simulink model "Katex_FullCar_R2017b_V03"  (R2026a)
settings: Solver=ode1  StopTime=1000  FixedStep=Ts  EnableMultiTasking=on
PostLoadFcn:
  | , if any(exist('dsrtsu_mdlpostloadfcn', 'file') == [2, 3, 6]), try dsrtsu_mdlpostloadfcn('Execute', bdroot); catch fprintf('Error in PostLoadFcn (dsrtsu_mdlpostloadfcn) for model "%s":\n %s\n', bdroot, lasterr); end, end,
  | , if any(exist('dsrtsu_mdlpostloadfcn', 'file') ~= 0), dsrtsu_mdlpostloadfcn('Execute', bdroot); end,
InitFcn:
  | , if any(exist('rtifpga_mdlclblib', 'file') ~= 0), rtifpga_mdlclblib('Init', bdroot); end,
  | 
  | 
  | init
undefined symbols (not defined in the file): locklim_sus, roundN, Ts
libraries: sl_discontinuities x29, simulink_extras x26, simulink x22, mjLib x1
(part 9 of 10)

== system Katex_FullCar_R2017b_V03/DGIST/_Low_Level_Ctrl/Steering_Low_Level_Controller/Torque Mode/Steering Motor Control3/Lag compensator(zeta)/Dot1 ==
  note: Dot
  in : Inport
  Sum1 : Sum  Inputs=+-  InputSameDT=on  SaturateOnIntegerOverflow=on  OutDataTypeStr=Inherit: Same as first input
  Sum2 : Sum  Inputs=+-  InputSameDT=on  SaturateOnIntegerOverflow=on  OutDataTypeStr=Inherit: Same as first input
  d : UnitDelay  SampleTime=Ts
  d1 : UnitDelay  SampleTime=Ts
  gain : Gain  Gain=2/Ts  SaturateOnIntegerOverflow=on  OutDataTypeStr=Inherit: Same as input  ParamDataTypeStr=Inherit: Same as input
  out : Outport  VectorParamsAs1DForOutWhenUnconnected=off
  wires:
  Sum1/1 -> d1/1, out/1
  d1/1 -> Sum1/2
  Sum2/1 -> gain/1
  in/1 -> d/1, Sum2/1
  d/1 -> Sum2/2
  gain/1 -> Sum1/1

== system Katex_FullCar_R2017b_V03/DGIST/_Low_Level_Ctrl/Steering_Low_Level_Controller/Torque Mode/Steering Motor Control3/Lag compensator(zeta)/a//(s+p) ==
  note: y(n) = [(2-p*Ts)*y(n-1)+a*Ts(u(n)+u(n-1))]/(2+p*Ts)
  note: H(s) = a/(s+p)
  note: s = 2/Ts*(z-1)/(z+1)
  In : Inport
  a : Inport  Port=2
  p : Inport  Port=3
  Constant : Constant  Value=2  SampleTime=Ts
  Product1 : Product  Inputs=*/  RndMeth=Zero
  Product11 : Product  RndMeth=Zero
  Product3 : Product  RndMeth=Zero
  Sum1 : Sum  Inputs=-+  InputSameDT=on  SaturateOnIntegerOverflow=on  OutDataTypeStr=Inherit: Same as first input
  Sum2 : Sum  InputSameDT=on  SaturateOnIntegerOverflow=on  OutDataTypeStr=Inherit: Same as first input
  Sum3 : Sum  InputSameDT=on  SaturateOnIntegerOverflow=on  OutDataTypeStr=Inherit: Same as first input
  Sum4 : Sum  InputSameDT=on  SaturateOnIntegerOverflow=on  OutDataTypeStr=Inherit: Same as first input
  d : UnitDelay  SampleTime=Ts
  d1 : UnitDelay  SampleTime=Ts
  gain : Gain  Gain=Ts  SaturateOnIntegerOverflow=on  OutDataTypeStr=Inherit: Same as input  ParamDataTypeStr=Inherit: Same as input
  gain1 : Gain  Gain=Ts  SaturateOnIntegerOverflow=on  OutDataTypeStr=Inherit: Same as input  ParamDataTypeStr=Inherit: Same as input
  Out : Outport  VectorParamsAs1DForOutWhenUnconnected=off
  wires:
  In/1 -> Sum3/1, d1/1
  d1/1 -> Sum3/2
  Sum3/1 -> gain/1
  Product11/1 -> Sum2/2
  Sum1/1 -> Product11/1
  Constant/1 -> Sum1/2, Sum4/2
  p/1 -> gain1/1
  gain1/1 -> Sum1/1, Sum4/1
  d/1 -> Product11/2
  Sum2/1 -> Product1/1
  Sum4/1 -> Product1/2
  Product1/1 -> Out/1, d/1
  gain/1 -> Product3/1
  a/1 -> Product3/2
  Product3/1 -> Sum2/1

== system Katex_FullCar_R2017b_V03/DGIST/_Low_Level_Ctrl/Suspension_Low_Level_Controller/Torque Mode/Subsystem/DOB(theta)/Dot ==
  note: Dot
  in : Inport
  Sum1 : Sum  Inputs=+-  InputSameDT=on  SaturateOnIntegerOverflow=on  OutDataTypeStr=Inherit: Same as first input
  Sum2 : Sum  Inputs=+-  InputSameDT=on  SaturateOnIntegerOverflow=on  OutDataTypeStr=Inherit: Same as first input
  d : UnitDelay  SampleTime=Ts
  d1 : UnitDelay  SampleTime=Ts
  gain : Gain  Gain=2/Ts  SaturateOnIntegerOverflow=on  OutDataTypeStr=Inherit: Same as input  ParamDataTypeStr=Inherit: Same as input
  out : Outport  VectorParamsAs1DForOutWhenUnconnected=off
  wires:
  Sum1/1 -> d1/1, out/1
  d1/1 -> Sum1/2
  Sum2/1 -> gain/1
  in/1 -> d/1, Sum2/1
  d/1 -> Sum2/2
  gain/1 -> Sum1/1

== system Katex_FullCar_R2017b_V03/DGIST/_Low_Level_Ctrl/Suspension_Low_Level_Controller/Torque Mode/Subsystem/DOB(theta)/Dot1 ==
  note: Dot
  in : Inport
  Sum1 : Sum  Inputs=+-  InputSameDT=on  SaturateOnIntegerOverflow=on  OutDataTypeStr=Inherit: Same as first input
  Sum2 : Sum  Inputs=+-  InputSameDT=on  SaturateOnIntegerOverflow=on  OutDataTypeStr=Inherit: Same as first input
  d : UnitDelay  SampleTime=Ts
  d1 : UnitDelay  SampleTime=Ts
  gain : Gain  Gain=2/Ts  SaturateOnIntegerOverflow=on  OutDataTypeStr=Inherit: Same as input  ParamDataTypeStr=Inherit: Same as input
  out : Outport  VectorParamsAs1DForOutWhenUnconnected=off
  wires:
  Sum1/1 -> d1/1, out/1
  d1/1 -> Sum1/2
  Sum2/1 -> gain/1
  in/1 -> d/1, Sum2/1
  d/1 -> Sum2/2
  gain/1 -> Sum1/1

== system Katex_FullCar_R2017b_V03/DGIST/_Low_Level_Ctrl/Suspension_Low_Level_Controller/Torque Mode/Subsystem/DOB(theta)/Dot2 ==
  note: Dot
  in : Inport
  Sum1 : Sum  Inputs=+-  InputSameDT=on  SaturateOnIntegerOverflow=on  OutDataTypeStr=Inherit: Same as first input
  Sum2 : Sum  Inputs=+-  InputSameDT=on  SaturateOnIntegerOverflow=on  OutDataTypeStr=Inherit: Same as first input
  d : UnitDelay  SampleTime=Ts
  d1 : UnitDelay  SampleTime=Ts
  gain : Gain  Gain=2/Ts  SaturateOnIntegerOverflow=on  OutDataTypeStr=Inherit: Same as input  ParamDataTypeStr=Inherit: Same as input
  out : Outport  VectorParamsAs1DForOutWhenUnconnected=off
  wires:
  Sum1/1 -> d1/1, out/1
  d1/1 -> Sum1/2
  Sum2/1 -> gain/1
  in/1 -> d/1, Sum2/1
  d/1 -> Sum2/2
  gain/1 -> Sum1/1

== system Katex_FullCar_R2017b_V03/DGIST/_Low_Level_Ctrl/Suspension_Low_Level_Controller/Torque Mode/Subsystem/DOB(theta)/Second order LPF ==
  note: y(n) = [Ts^2*w^2*{x(n)+2*x(n-1)+x(n-2)}-(2*w^2*Ts^2-8)*y(n-1)-(4+w^2*Ts^2+2*zeta*Ts*w)*y(n-2)]
      | /(4+w^2*Ts^2+2*zeta*Ts*w)
  note: H(s) = w^2/(s^2+2*zeta*w*s+w^2)
  note: s = 2/Ts*(z-1)/(z+1)
  In : Inport
  fc : Inport  Port=2
  zeta : Inport  Port=3
  Constant : Constant  Value=Ts  SampleTime=Ts
  Constant1 : Constant  Value=8  SampleTime=Ts
  Constant2 : Constant  Value=4  SampleTime=Ts
  Delay : Delay  InitialCondition=0  SampleTime=Ts
  Delay1 : Delay  DelayLength=1  InitialCondition=0  SampleTime=Ts
  Delay2 : Delay  DelayLength=1  InitialCondition=0  SampleTime=Ts
  Delay3 : Delay  InitialCondition=0  SampleTime=Ts
  Product1 : Product  Inputs=*/  RndMeth=Zero
  Product2 : Product  Inputs=4  RndMeth=Zero
  Product3 : Product  RndMeth=Zero
  Product4 : Product  RndMeth=Zero
  Sum1 : Sum  Inputs=+-  InputSameDT=on  SaturateOnIntegerOverflow=on  OutDataTypeStr=Inherit: Same as first input
  Sum2 : Sum  Inputs=+-  InputSameDT=on  SaturateOnIntegerOverflow=on  OutDataTypeStr=Inherit: Same as first input
  Sum3 : Sum  Inputs=+++  InputSameDT=on  SaturateOnIntegerOverflow=on  OutDataTypeStr=Inherit: Same as first input
  Sum4 : Sum  Inputs=+-  InputSameDT=on  SaturateOnIntegerOverflow=on  OutDataTypeStr=Inherit: Same as first input
  Sum5 : Sum  Inputs=+-+  InputSameDT=on  SaturateOnIntegerOverflow=on  OutDataTypeStr=Inherit: Same as first input
  Sum6 : Sum  Inputs=+++  InputSameDT=on  SaturateOnIntegerOverflow=on  OutDataTypeStr=Inherit: Same as first input
  gain1 : Gain  Gain=2  SaturateOnIntegerOverflow=on  OutDataTypeStr=Inherit: Same as input  ParamDataTypeStr=Inherit: Same as input
  gain2 : Gain  Gain=2*pi  SaturateOnIntegerOverflow=on  OutDataTypeStr=Inherit: Same as input  ParamDataTypeStr=Inherit: Same as input
  gain3 : Gain  Gain=2  SaturateOnIntegerOverflow=on  OutDataTypeStr=Inherit: Same as input  ParamDataTypeStr=Inherit: Same as input
  gain4 : Gain  Gain=4  SaturateOnIntegerOverflow=on  OutDataTypeStr=Inherit: Same as input  ParamDataTypeStr=Inherit: Same as input
  "x(n), x(n-1), x(n-2)" : Product  RndMeth=Zero
  y(n-1) : Product  RndMeth=Zero
  y(n-2) : Product  RndMeth=Zero
  Dist_hat : Outport  VectorParamsAs1DForOutWhenUnconnected=off
  wires:
  Product1/1 -> Dist_hat/1, Delay3/1, Delay2/1
  Sum2/1 -> Product1/1
  fc/1 -> gain2/1
  In/1 -> Delay1/1, Delay/1, Sum3/1
  gain2/1 -> Product3/1, Product2/2, Product2/1
  Constant/1 -> Product3/2, Product2/4, Product2/3
  Delay1/1 -> gain1/1
  gain1/1 -> Sum3/2
  Delay/1 -> Sum3/3
  Sum3/1 -> "x(n), x(n-1), x(n-2)"/1
  Product2/1 -> Sum5/1, Sum6/1, "x(n), x(n-1), x(n-2)"/2, gain3/1
  "x(n), x(n-1), x(n-2)"/1 -> Sum1/1
  Sum1/1 -> Sum2/1
  y(n-1)/1 -> Sum1/2
  Sum4/1 -> y(n-1)/1
  gain3/1 -> Sum4/1
  Constant1/1 -> Sum4/2
  Delay2/1 -> y(n-1)/2
  Product3/1 -> gain4/1
  Constant2/1 -> Sum5/3, Sum6/3
  Sum5/1 -> y(n-2)/1
  Delay3/1 -> y(n-2)/2
  y(n-2)/1 -> Sum2/2
  Sum6/1 -> Product1/2
  zeta/1 -> Product4/2
  gain4/1 -> Product4/1
  Product4/1 -> Sum6/2, Sum5/2

== system Katex_FullCar_R2017b_V03/DGIST/_Low_Level_Ctrl/Suspension_Low_Level_Controller/Torque Mode/Subsystem/Feedforward(theta)/Dot ==
  note: Dot
  in : Inport
  Sum1 : Sum  Inputs=+-  InputSameDT=on  SaturateOnIntegerOverflow=on  OutDataTypeStr=Inherit: Same as first input
  Sum2 : Sum  Inputs=+-  InputSameDT=on  SaturateOnIntegerOverflow=on  OutDataTypeStr=Inherit: Same as first input
  d : UnitDelay  SampleTime=Ts
  d1 : UnitDelay  SampleTime=Ts
  gain : Gain  Gain=2/Ts  SaturateOnIntegerOverflow=on  OutDataTypeStr=Inherit: Same as input  ParamDataTypeStr=Inherit: Same as input
  out : Outport  VectorParamsAs1DForOutWhenUnconnected=off
  wires:
  Sum1/1 -> d1/1, out/1
  d1/1 -> Sum1/2
  Sum2/1 -> gain/1
  in/1 -> d/1, Sum2/1
  d/1 -> Sum2/2
  gain/1 -> Sum1/1

== system Katex_FullCar_R2017b_V03/DGIST/_Low_Level_Ctrl/Suspension_Low_Level_Controller/Torque Mode/Subsystem/Feedforward(theta)/Dot1 ==
  note: Dot
  in : Inport
  Sum1 : Sum  Inputs=+-  InputSameDT=on  SaturateOnIntegerOverflow=on  OutDataTypeStr=Inherit: Same as first input
  Sum2 : Sum  Inputs=+-  InputSameDT=on  SaturateOnIntegerOverflow=on  OutDataTypeStr=Inherit: Same as first input
  d : UnitDelay  SampleTime=Ts
  d1 : UnitDelay  SampleTime=Ts
  gain : Gain  Gain=2/Ts  SaturateOnIntegerOverflow=on  OutDataTypeStr=Inherit: Same as input  ParamDataTypeStr=Inherit: Same as input
  out : Outport  VectorParamsAs1DForOutWhenUnconnected=off
  wires:
  Sum1/1 -> d1/1, out/1
  d1/1 -> Sum1/2
  Sum2/1 -> gain/1
  in/1 -> d/1, Sum2/1
  d/1 -> Sum2/2
  gain/1 -> Sum1/1

== system Katex_FullCar_R2017b_V03/DGIST/_Low_Level_Ctrl/Suspension_Low_Level_Controller/Torque Mode/Subsystem/Feedforward(theta)/Dot2 ==
  note: Dot
  in : Inport
  Sum1 : Sum  Inputs=+-  InputSameDT=on  SaturateOnIntegerOverflow=on  OutDataTypeStr=Inherit: Same as first input
  Sum2 : Sum  Inputs=+-  InputSameDT=on  SaturateOnIntegerOverflow=on  OutDataTypeStr=Inherit: Same as first input
  d : UnitDelay  SampleTime=Ts
  d1 : UnitDelay  SampleTime=Ts
  gain : Gain  Gain=2/Ts  SaturateOnIntegerOverflow=on  OutDataTypeStr=Inherit: Same as input  ParamDataTypeStr=Inherit: Same as input
  out : Outport  VectorParamsAs1DForOutWhenUnconnected=off
  wires:
  Sum1/1 -> d1/1, out/1
  d1/1 -> Sum1/2
  Sum2/1 -> gain/1
  in/1 -> d/1, Sum2/1
  d/1 -> Sum2/2
  gain/1 -> Sum1/1

== system Katex_FullCar_R2017b_V03/DGIST/_Low_Level_Ctrl/Suspension_Low_Level_Controller/Torque Mode/Subsystem/Feedforward(theta)/Second order LPF ==
  note: y(n) = [Ts^2*w^2*{x(n)+2*x(n-1)+x(n-2)}-(2*w^2*Ts^2-8)*y(n-1)-(4+w^2*Ts^2+2*zeta*Ts*w)*y(n-2)]
      | /(4+w^2*Ts^2+2*zeta*Ts*w)
  note: H(s) = w^2/(s^2+2*zeta*w*s+w^2)
  note: s = 2/Ts*(z-1)/(z+1)
  In : Inport
  fc : Inport  Port=2
  zeta : Inport  Port=3
  Constant : Constant  Value=Ts  SampleTime=Ts
  Constant1 : Constant  Value=8  SampleTime=Ts
  Constant2 : Constant  Value=4  SampleTime=Ts
  Delay : Delay  InitialCondition=0  SampleTime=Ts
  Delay1 : Delay  DelayLength=1  InitialCondition=0  SampleTime=Ts
  Delay2 : Delay  DelayLength=1  InitialCondition=0  SampleTime=Ts
  Delay3 : Delay  InitialCondition=0  SampleTime=Ts
  Product1 : Product  Inputs=*/  RndMeth=Zero
  Product2 : Product  Inputs=4  RndMeth=Zero
  Product3 : Product  RndMeth=Zero
  Product4 : Product  RndMeth=Zero
  Sum1 : Sum  Inputs=+-  InputSameDT=on  SaturateOnIntegerOverflow=on  OutDataTypeStr=Inherit: Same as first input
  Sum2 : Sum  Inputs=+-  InputSameDT=on  SaturateOnIntegerOverflow=on  OutDataTypeStr=Inherit: Same as first input
  Sum3 : Sum  Inputs=+++  InputSameDT=on  SaturateOnIntegerOverflow=on  OutDataTypeStr=Inherit: Same as first input
  Sum4 : Sum  Inputs=+-  InputSameDT=on  SaturateOnIntegerOverflow=on  OutDataTypeStr=Inherit: Same as first input
  Sum5 : Sum  Inputs=+-+  InputSameDT=on  SaturateOnIntegerOverflow=on  OutDataTypeStr=Inherit: Same as first input
  Sum6 : Sum  Inputs=+++  InputSameDT=on  SaturateOnIntegerOverflow=on  OutDataTypeStr=Inherit: Same as first input
  gain1 : Gain  Gain=2  SaturateOnIntegerOverflow=on  OutDataTypeStr=Inherit: Same as input  ParamDataTypeStr=Inherit: Same as input
  gain2 : Gain  Gain=2*pi  SaturateOnIntegerOverflow=on  OutDataTypeStr=Inherit: Same as input  ParamDataTypeStr=Inherit: Same as input
  gain3 : Gain  Gain=2  SaturateOnIntegerOverflow=on  OutDataTypeStr=Inherit: Same as input  ParamDataTypeStr=Inherit: Same as input
  gain4 : Gain  Gain=4  SaturateOnIntegerOverflow=on  OutDataTypeStr=Inherit: Same as input  ParamDataTypeStr=Inherit: Same as input
  "x(n), x(n-1), x(n-2)" : Product  RndMeth=Zero
  y(n-1) : Product  RndMeth=Zero
  y(n-2) : Product  RndMeth=Zero
  Out : Outport  VectorParamsAs1DForOutWhenUnconnected=off
  wires:
  Product1/1 -> Out/1, Delay3/1, Delay2/1
  Sum2/1 -> Product1/1
  fc/1 -> gain2/1
  In/1 -> Delay1/1, Delay/1, Sum3/1
  gain2/1 -> Product3/1, Product2/2, Product2/1
  Constant/1 -> Product3/2, Product2/4, Product2/3
  Delay1/1 -> gain1/1
  gain1/1 -> Sum3/2
  Delay/1 -> Sum3/3
  Sum3/1 -> "x(n), x(n-1), x(n-2)"/1
  Product2/1 -> Sum5/1, Sum6/1, "x(n), x(n-1), x(n-2)"/2, gain3/1
  "x(n), x(n-1), x(n-2)"/1 -> Sum1/1
  Sum1/1 -> Sum2/1
  y(n-1)/1 -> Sum1/2
  Sum4/1 -> y(n-1)/1
  gain3/1 -> Sum4/1
  Constant1/1 -> Sum4/2
  Delay2/1 -> y(n-1)/2
  Product3/1 -> gain4/1
  Constant2/1 -> Sum5/3, Sum6/3
  Sum5/1 -> y(n-2)/1
  Delay3/1 -> y(n-2)/2
  y(n-2)/1 -> Sum2/2
  Sum6/1 -> Product1/2
  zeta/1 -> Product4/2
  gain4/1 -> Product4/1
  Product4/1 -> Sum6/2, Sum5/2

== system Katex_FullCar_R2017b_V03/DGIST/_Low_Level_Ctrl/Suspension_Low_Level_Controller/Torque Mode/Subsystem/Lag compensator(zeta)/Dot1 ==
  note: Dot
  in : Inport
  Sum1 : Sum  Inputs=+-  InputSameDT=on  SaturateOnIntegerOverflow=on  OutDataTypeStr=Inherit: Same as first input
  Sum2 : Sum  Inputs=+-  InputSameDT=on  SaturateOnIntegerOverflow=on  OutDataTypeStr=Inherit: Same as first input
  d : UnitDelay  SampleTime=Ts
  d1 : UnitDelay  SampleTime=Ts
  gain : Gain  Gain=2/Ts  SaturateOnIntegerOverflow=on  OutDataTypeStr=Inherit: Same as input  ParamDataTypeStr=Inherit: Same as input
  out : Outport  VectorParamsAs1DForOutWhenUnconnected=off
  wires:
  Sum1/1 -> d1/1, out/1
  d1/1 -> Sum1/2
  Sum2/1 -> gain/1
  in/1 -> d/1, Sum2/1
  d/1 -> Sum2/2
  gain/1 -> Sum1/1

== system Katex_FullCar_R2017b_V03/DGIST/_Low_Level_Ctrl/Suspension_Low_Level_Controller/Torque Mode/Subsystem/Lag compensator(zeta)/a//(s+p) ==
  note: y(n) = [(2-p*Ts)*y(n-1)+a*Ts(u(n)+u(n-1))]/(2+p*Ts)
  note: H(s) = a/(s+p)
  note: s = 2/Ts*(z-1)/(z+1)
  In : Inport
  a : Inport  Port=2
  p : Inport  Port=3
  Constant : Constant  Value=2  SampleTime=Ts
  Product1 : Product  Inputs=*/  RndMeth=Zero
  Product11 : Product  RndMeth=Zero
  Product3 : Product  RndMeth=Zero
  Sum1 : Sum  Inputs=-+  InputSameDT=on  SaturateOnIntegerOverflow=on  OutDataTypeStr=Inherit: Same as first input
  Sum2 : Sum  InputSameDT=on  SaturateOnIntegerOverflow=on  OutDataTypeStr=Inherit: Same as first input
  Sum3 : Sum  InputSameDT=on  SaturateOnIntegerOverflow=on  OutDataTypeStr=Inherit: Same as first input
  Sum4 : Sum  InputSameDT=on  SaturateOnIntegerOverflow=on  OutDataTypeStr=Inherit: Same as first input
  d : UnitDelay  SampleTime=Ts
  d1 : UnitDelay  SampleTime=Ts
  gain : Gain  Gain=Ts  SaturateOnIntegerOverflow=on  OutDataTypeStr=Inherit: Same as input  ParamDataTypeStr=Inherit: Same as input
  gain1 : Gain  Gain=Ts  SaturateOnIntegerOverflow=on  OutDataTypeStr=Inherit: Same as input  ParamDataTypeStr=Inherit: Same as input
  Out : Outport  VectorParamsAs1DForOutWhenUnconnected=off
  wires:
  In/1 -> Sum3/1, d1/1
  d1/1 -> Sum3/2
  Sum3/1 -> gain/1
  Product11/1 -> Sum2/2
  Sum1/1 -> Product11/1
  Constant/1 -> Sum1/2, Sum4/2
  p/1 -> gain1/1
  gain1/1 -> Sum1/1, Sum4/1
  d/1 -> Product11/2
  Sum2/1 -> Product1/1
  Sum4/1 -> Product1/2
  Product1/1 -> Out/1, d/1
  gain/1 -> Product3/1
  a/1 -> Product3/2
  Product3/1 -> Sum2/1

== system Katex_FullCar_R2017b_V03/DGIST/_Low_Level_Ctrl/Suspension_Low_Level_Controller/Torque Mode/Subsystem/Sus Ref Mode/If Action Subsystem ==
  In1 : Inport
  Action Port : ActionPort  ActionPortLabel=if(u1 == 0 )
  Out1 : Outport  VectorParamsAs1DForOutWhenUnconnected=off
  wires:
  In1/1 -> Out1/1

== system Katex_FullCar_R2017b_V03/DGIST/_Low_Level_Ctrl/Suspension_Low_Level_Controller/Torque Mode/Subsystem/Sus Ref Mode/If Action Subsystem1 ==
  In1 : Inport
  Action Port : ActionPort  ActionPortLabel=elseif(u1 ==1)
  Out1 : Outport  VectorParamsAs1DForOutWhenUnconnected=off
  wires:
  In1/1 -> Out1/1

== system Katex_FullCar_R2017b_V03/DGIST/_Low_Level_Ctrl/Suspension_Low_Level_Controller/Torque Mode/Subsystem/Sus Ref Mode/If Action Subsystem2 ==
  In1 : Inport
  Action Port : ActionPort  ActionPortLabel=else
  Out1 : Outport  VectorParamsAs1DForOutWhenUnconnected=off
  wires:
  In1/1 -> Out1/1

== system Katex_FullCar_R2017b_V03/MuJoCo Interface/FL_Motor_Control/Drv_Driver/Velocity Mode/FL_vel_velocity_motor_driver/poleplacement(PI)1/Integ ==
  error : Inport
  Add1 : Sum
  Add2 : Sum
  Delay : Delay  DelayLength=1  SampleTime=Ts
  Delay1 : Delay  DelayLength=1  SampleTime=Ts
  Gain2 : Gain  Gain=Ts/2
  Out1 : Outport
  wires:
  Gain2/1 -> Add2/1
  Add1/1 -> Gain2/1
  Delay1/1 -> Add2/2
  Add2/1 -> Delay1/1, Out1/1
  Delay/1 -> Add1/1
  error/1 -> Add1/2, Delay/1

== system Katex_FullCar_R2017b_V03/MuJoCo Interface/FL_Motor_Control/Sus_Driver/Position Mode/FL_sus_position_motor_driver/poleplacement(PD)+I/Integ ==
  error : Inport
  Add1 : Sum
  Add2 : Sum
  Delay : Delay  DelayLength=1  SampleTime=Ts
  Delay1 : Delay  DelayLength=1  SampleTime=Ts
  Gain2 : Gain  Gain=Ts/2
  Out1 : Outport
  wires:
  error/1 -> Delay/1, Add1/2
  Delay/1 -> Add1/1
  Add2/1 -> Out1/1, Delay1/1
  Delay1/1 -> Add2/2
  Add1/1 -> Gain2/1
  Gain2/1 -> Add2/1

== system Katex_FullCar_R2017b_V03/MuJoCo Interface/FR_Motor_Control/Drv_Driver/Velocity Mode/FR_vel_velocity_motor_driver/poleplacement(PI)1/Integ ==
  error : Inport
  Add1 : Sum
  Add2 : Sum
  Delay : Delay  DelayLength=1  SampleTime=Ts
  Delay1 : Delay  DelayLength=1  SampleTime=Ts
  Gain2 : Gain  Gain=Ts/2
  Out1 : Outport
  wires:
  error/1 -> Delay/1, Add1/2
  Delay/1 -> Add1/1
  Add2/1 -> Out1/1, Delay1/1
  Delay1/1 -> Add2/2
  Add1/1 -> Gain2/1
  Gain2/1 -> Add2/1

== system Katex_FullCar_R2017b_V03/MuJoCo Interface/FR_Motor_Control/Sus_Driver/Position Mode/FR_sus_position_motor_driver/poleplacement(PD)+I/Integ ==
  error : Inport
  Add1 : Sum
  Add2 : Sum
  Delay : Delay  DelayLength=1  SampleTime=Ts
  Delay1 : Delay  DelayLength=1  SampleTime=Ts
  Gain2 : Gain  Gain=Ts/2
  Out1 : Outport
  wires:
  Gain2/1 -> Add2/1
  Add1/1 -> Gain2/1
  Delay1/1 -> Add2/2
  Add2/1 -> Delay1/1, Out1/1
  Delay/1 -> Add1/1
  error/1 -> Add1/2, Delay/1

== system Katex_FullCar_R2017b_V03/MuJoCo Interface/RL_Motor_Control/Drv_Driver/Velocity Mode/RL_vel_velocity_motor_driver/poleplacement(PI)1/Integ ==
  error : Inport
  Add1 : Sum
  Add2 : Sum
  Delay : Delay  DelayLength=1  SampleTime=Ts
  Delay1 : Delay  DelayLength=1  SampleTime=Ts
  Gain2 : Gain  Gain=Ts/2
  Out1 : Outport
  wires:
  error/1 -> Delay/1, Add1/2
  Delay/1 -> Add1/1
  Add2/1 -> Out1/1, Delay1/1
  Delay1/1 -> Add2/2
  Add1/1 -> Gain2/1
  Gain2/1 -> Add2/1

== system Katex_FullCar_R2017b_V03/MuJoCo Interface/RL_Motor_Control/Sus_Driver/Position Mode/RL_sus_position_motor_driver/poleplacement(PD)+I/Integ ==
  error : Inport
  Add1 : Sum
  Add2 : Sum
  Delay : Delay  DelayLength=1  SampleTime=Ts
  Delay1 : Delay  DelayLength=1  SampleTime=Ts
  Gain2 : Gain  Gain=Ts/2
  Out1 : Outport
  wires:
  Gain2/1 -> Add2/1
  Add1/1 -> Gain2/1
  Delay1/1 -> Add2/2
  Add2/1 -> Delay1/1, Out1/1
  Delay/1 -> Add1/1
  error/1 -> Add1/2, Delay/1

== system Katex_FullCar_R2017b_V03/MuJoCo Interface/RR_Motor_Control/Drv_Driver/Velocity Mode/RR_vel_velocity_motor_driver/poleplacement(PI)1/Integ ==
  error : Inport
  Add1 : Sum
  Add2 : Sum
  Delay : Delay  DelayLength=1  SampleTime=Ts
  Delay1 : Delay  DelayLength=1  SampleTime=Ts
  Gain2 : Gain  Gain=Ts/2
  Out1 : Outport
  wires:
  error/1 -> Delay/1, Add1/2
  Delay/1 -> Add1/1
  Add2/1 -> Out1/1, Delay1/1
  Delay1/1 -> Add2/2
  Add1/1 -> Gain2/1
  Gain2/1 -> Add2/1

== system Katex_FullCar_R2017b_V03/MuJoCo Interface/RR_Motor_Control/Sus_Driver/Position Mode/RR_sus_position_motor_driver/poleplacement(PD)+I/Integ ==
  error : Inport
  Add1 : Sum
  Add2 : Sum
  Delay : Delay  DelayLength=1  SampleTime=Ts
  Delay1 : Delay  DelayLength=1  SampleTime=Ts
  Gain2 : Gain  Gain=Ts/2
  Out1 : Outport
  wires:
  Gain2/1 -> Add2/1
  Add1/1 -> Gain2/1
  Delay1/1 -> Add2/2
  Add2/1 -> Delay1/1, Out1/1
  Delay/1 -> Add1/1
  error/1 -> Add1/2, Delay/1

== matlab function Katex_FullCar_R2017b_V03/DGIST/_High_Level_Ctrl/Orientation_Pos_Ctrl/MATLAB Function ==
  data: Roll_ref input; SusPos_ref output; Pitch_ref input; SusPos_neutral input; RobotWidth input; RobotLength input; SusLinkLength input; SusPosLimit input
function SusPos_ref = Orientation_Position_Mapping( ...
    Roll_ref, Pitch_ref, SusPos_neutral, ...
    RobotWidth, RobotLength, SusLinkLength, SusPosLimit)
%#codegen
% Output order: FL, FR, RL, RR
% Angle unit: rad
% Length unit: m

% Coordinate:
% +x     : forward
% +y     : vehicle left
% +z     : upward
% +Roll  : vehicle left chassis moves upward
% +Pitch : vehicle front chassis moves downward

% Suspension:
% SusPos_ref > 0 : suspension moves upward
% SusPos_ref < 0 : suspension moves downward

% Parameter 오류 시 중립 위치 유지
SusPos_ref = SusPos_neutral;

if RobotWidth < 0 || RobotLength <= 0 || ...
        SusLinkLength <= 0 || SusPosLimit <= 0
    return;
end

% Wheel order: FL, FR, RL, RR
roll_sign  = [ -1.0; 1.0;  -1.0; 1.0];
pitch_sign = [1.0; 1.0;  -1.0;  -1.0];

for i = 1:4

    % Roll/ Pitch 에 의한 chassis corner 수직 변위 [m]
    h_body = ...
        roll_sign(i)*(RobotWidth/2.0)*sin(Roll_ref) ...
        + pitch_sign(i)*(RobotLength/2.0)*sin(Pitch_ref);

    % Wheel 위치가 지면에 고정되어 있다고 가정
    %
    % h_body
    % + L*sin(q + roll_sign*Roll)
    % = L*sin(q_neutral)
    asin_input = ...
        sin(SusPos_neutral(i)) ...
        - h_body/SusLinkLength;

    % asin 입력 범위 보호
    if asin_input > 1.0
        asin_input = 1.0;
    elseif asin_input < -1.0
        asin_input = -1.0;
    end

    % Suspension load-side 절대 위치지령 [rad]
    SusPos_ref(i) = ...
        asin(asin_input) ...
        - roll_sign(i)*Roll_ref;

    % Load-side position saturation [rad]
    if SusPos_ref(i) > SusPosLimit
        SusPos_ref(i) = SusPosLimit;
    elseif SusPos_ref(i) < -SusPosLimit
        SusPos_ref(i) = -SusPosLimit;
    end
end
end

== matlab function Katex_FullCar_R2017b_V03/DGIST/Attitude&Force distribution opt/Desired Height, Roll, Pitch Caculate/MATLAB Function ==
  data: u input; y output; roll input; pitch input; sus_ang_fl input; sus_ang_fr input; sus_ang_rl input; sus_ang_rr input; v output
function [y,v] = fcn(u, roll, pitch, sus_ang_fl, sus_ang_fr, sus_ang_rl, sus_ang_rr)

%% Input Setting
desired_attitude = zeros(3,1);
R = roll;
P = pitch;
Afl = deg2rad(sus_ang_fl);
Afr = deg2rad(sus_ang_fr);
Arl = deg2rad(sus_ang_rl);
Arr = deg2rad(sus_ang_rr);
A = [Afl,Afr,Arl,Arr];

for i = 1:3
    desired_attitude(i)=u(i);
end

DA = desired_attitude;

%% Output Setting
error = zeros(3,1);

%% Robot 
sus_link = 0.16;
trunk_width = 0.42;
trunk_length = 1.08 ; 
base_com_2_sus_vertical_length = 0.076193-0.04; % 트렁크 좌표계에서 샤시 com 높이 0.076193, 서스펜션 조인트 높이 0.04
x_sign = [1, 1, -1, -1];
y_sign = [1, -1, 1, -1];
wheel_point_matrix = zeros(4,4);

for i = 1:4
    x = x_sign(i)*(trunk_length/2);
    y = y_sign(i)*(trunk_width/2 + sus_link*cos(A(i)));
    z = -base_com_2_sus_vertical_length + sus_link*sin(A(i));
    wheel_point_matrix(i,:) = [1, x, y, z];
end


%% Height calculate
% plane calculate 
% 평면: a + b*x + c*y + z = 0
% 정리: a + b*x + c*y = -z

M = wheel_point_matrix(:,1:3); % 네 바퀴의 [1, x, y]
rhs = -wheel_point_matrix(:,4); % 네 바퀴의 -z

plane = M\rhs; % [a ; b ; c]

height = plane(1);

% error

error(1) = DA(1)-height; %[m]
error(2) = DA(2) - R;    %[deg]
error(3) = DA(3) - P;    %[deg]



y = error;
v= u(4);
end

== matlab function Katex_FullCar_R2017b_V03/DGIST/Attitude&Force distribution opt/Desired Wrench(PID)/MATLAB Function ==
  data: error input; y output; Kp input; Ki input; Kd input; Ts input; fc input; y_min input; y_max input
function y = fcn(error, Kp, Ki, Kd, Ts, fc, y_min, y_max)
%#codegen
%
% 입력: 아래 벡터는 모두 3x1
% error = [height 오차(m); roll 오차(deg); pitch 오차(deg)]
% Kp, Ki, Kd = [height gain; roll gain; pitch gain]
%
% y_min = [추가 수직 힘 하한(N);
%          roll 모멘트 하한(Nm);
%          pitch 모멘트 하한(Nm)]
%
% y_max = [추가 수직 힘 상한(N);
%          roll 모멘트 상한(Nm);
%          pitch 모멘트 상한(Nm)]
%
% Ts : 실제 제어기 실행 주기 [s]
% fc : 미분 필터 차단 주파수 [Hz]
%
% 출력
% y = [추가 수직 힘(N); roll 모멘트(Nm); pitch 모멘트(Nm)]

%% 입력 조건
assert(Ts > 0 && isfinite(Ts), 'Ts must be positive and finite.');
assert(fc > 0 && isfinite(fc), 'fc must be positive and finite.');
assert(all(y_min <= y_max), 'Invalid output limits.');

%% 이전 값 저장
persistent error_prev integral derivative_prev
persistent integral_input_prev saturation_error_prev

if isempty(error_prev)
    error_prev = error;
    integral = zeros(3,1);
    derivative_prev = zeros(3,1);

    integral_input_prev = error;
    saturation_error_prev = zeros(3,1);
end

%% 미분 필터 계수
tau = 1 / (2*pi*fc);

alpha = (2*tau - Ts) / (2*tau + Ts);
beta  = 2 / (2*tau + Ts);

%% PID 계산
y = zeros(3,1);
derivative = zeros(3,1);

for i = 1:3

    %% P
    P = Kp(i) * error(i);

    %% Anti-windup gain
    if Kp(i) ~= 0
        Kaw = 1 / Kp(i);
    else
        % Kp=0이면 역수를 정의할 수 없으므로 보정 비활성화
        Kaw = 0;
    end

    %% I: anti-windup이 반영된 오차를 적분
    if Ki(i) ~= 0

        % 이전 샘플의 포화 차이를 피드백
        integral_input = error(i) ...
            + Kaw * saturation_error_prev(i);

        % 사다리꼴 적분
        integral(i) = integral(i) ...
            + Ts/2 * (integral_input ...
                      + integral_input_prev(i));

        integral_input_prev(i) = integral_input;

    else

        integral(i) = 0;
        integral_input_prev(i) = error(i);

    end

    I = Ki(i) * integral(i);

    %% D: 저역통과 필터가 포함된 오차 미분
    derivative(i) = alpha * derivative_prev(i) ...
        + beta * (error(i) - error_prev(i));

    D = Kd(i) * derivative(i);

    %% 포화 적용 전 출력
    y_raw = P + I + D;

    %% 출력 saturation
    y(i) = min(max(y_raw, y_min(i)), y_max(i));

    %% 다음 샘플에서 사용할 포화 차이
    if Ki(i) ~= 0
        saturation_error_prev(i) = y(i) - y_raw;
    else
        saturation_error_prev(i) = 0;
    end

end

%% 다음 계산을 위해 저장
error_prev = error;
derivative_prev = derivative;

end

== matlab function Katex_FullCar_R2017b_V03/DGIST/Attitude_reference_generator/MATLAB Function ==
  data: u input; y output
function y = fcn(u)

%% Input Setting
Afl = deg2rad(u(1));
Afr = deg2rad(u(2));
Arl = deg2rad(u(3));
Arr = deg2rad(u(4));
A = [Afl,Afr,Arl,Arr];


%% Robot 
sus_link = 0.16;
trunk_width = 0.42;
trunk_length = 1.08 ; 
base_com_2_sus_vertical_length = 0.076193-0.04; % 트렁크 좌표계에서 샤시 com 높이 0.076193, 서스펜션 조인트 높이 0.04
x_sign = [1, 1, -1, -1];
y_sign = [1, -1, 1, -1];
sus_point_matrix = zeros(4,4);

for i = 1:4
    x = x_sign(i)*(trunk_length/2);
    y = y_sign(i)*(trunk_width/2 + sus_link*cos(A(i)));
    z = -base_com_2_sus_vertical_length + sus_link*sin(A(i));
    sus_point_matrix(i,:) = [1, x, y, z];
end


%% Height calculate
% plane calculate 
% 평면: a + b*x + c*y + z = 0
% 정리: a + b*x + c*y = -z

M = sus_point_matrix(:,1:3); % 네 바퀴의 [1, x, y]
rhs = -sus_point_matrix(:,4); % 네 바퀴의 -z

plane = M\rhs; % [a ; b ; c]

height = plane(1);

y = height;

end

== matlab function Katex_FullCar_R2017b_V03/DGIST/Attitude&Force distribution opt/AX=b, QP/MATLAB Function ==
  data: u input; y output; sus_ang_fl input; sus_ang_fr input; sus_ang_rl input; sus_ang_rr input
function y = fcn(u,sus_ang_fl, sus_ang_fr, sus_ang_rl, sus_ang_rr)
%#codegen
%
% 입력
% u = [추가 수직 힘(N); roll 모멘트(Nm); pitch 모멘트(Nm)]
% sus_ang_* : deg
%
% 출력
% y = [Fz_FL; Fz_FR; Fz_RL; Fz_RR] [N]
%
% 좌표계: 샤시 COM 원점, x 전방, y 좌측, z 위쪽
% 가정: 조향각 0도, cover 각도 = -sus 각도

%% Input Setting
theta = deg2rad([sus_ang_fl; sus_ang_fr; ...
                sus_ang_rl; sus_ang_rr]);

desired_wrench = [u(1); u(2); u(3)];

assert(all(isfinite(theta)), 'Suspension angle is not finite.');
assert(all(isfinite(desired_wrench)), 'Desired wrench is not finite.');

%% Robot geometry [m]
sus_link = 0.16;

trunk_width  = 0.42;
trunk_length = 1.08;

base_com_2_sus_vertical_length = 0.076193 - 0.04;

wheel_offset_x = 0.005;
wheel_offset_y = 0.193;
wheel_offset_z = 0.05;

% FL, FR, RL, RR
x_sign = [1;  1; -1; -1];
y_sign = [1; -1;  1; -1];

%% Mass and gravity
chassis_mass = 15.0;   % 샤시 [kg]
sus_mass     = 2.5;    % 각 코너, 휠 제외 [kg]
wheel_mass   = 5.0;    % 각 휠 [kg]

gravity = 1.67;        % 현재 XML 중력 크기 [m/s^2]

total_mass = chassis_mass + 4*sus_mass + 4*wheel_mass;

%% COM and wheel-center positions
base_com = zeros(3,1);
sus_com = zeros(3,4);
wheel_center = zeros(3,4);

for i = 1:4

    % 서스펜션 조인트 위치: 샤시 COM 기준
    joint_x = x_sign(i) * trunk_length/2;
    joint_y = y_sign(i) * trunk_width/2;
    joint_z = -base_com_2_sus_vertical_length;

    % 서스펜션 lumped COM: 링크 길이의 1/2 지점
    sus_com(1,i) = joint_x;

    sus_com(2,i) = joint_y ...
        + y_sign(i) * (sus_link/2) * cos(theta(i));

    sus_com(3,i) = joint_z ...
        + (sus_link/2) * sin(theta(i));

    % 휠 중심
    wheel_center(1,i) = joint_x ...
        + x_sign(i) * wheel_offset_x;

    wheel_center(2,i) = joint_y ...
        + y_sign(i) * ...
        (sus_link*cos(theta(i)) + wheel_offset_y);

    wheel_center(3,i) = joint_z ...
        + sus_link*sin(theta(i)) - wheel_offset_z;

end

%% Gravity compensation wrench
% 총 9개 점: 샤시 1개 + 서스펜션 4개 + 휠 4개
points = [base_com, sus_com, wheel_center];

masses = [chassis_mass, ...
          sus_mass, sus_mass, sus_mass, sus_mass, ...
          wheel_mass, wheel_mass, wheel_mass, wheel_mass];

gravity_wrench = zeros(3,1);

for i = 1:9

    weight = masses(i) * gravity;

    px = points(1,i);
    py = points(2,i);

    % 중력을 지지하기 위해 필요한 위쪽 힘과 모멘트
    gravity_wrench(1) = gravity_wrench(1) + weight;
    gravity_wrench(2) = gravity_wrench(2) + py*weight;
    gravity_wrench(3) = gravity_wrench(3) - px*weight;

end

%% A matrix
% A * Fz = [전체 수직 힘; roll 모멘트; pitch 모멘트]
A = zeros(3,4);

for i = 1:4

    px = wheel_center(1,i);
    py = wheel_center(2,i);

    A(:,i) = [1; py; -px];

end

%% Target wrench
b = gravity_wrench + desired_wrench;

%% Force bounds [N]
fz_min = 0.0;
fz_max = 100.0;    % 예시 상한: 실제 허용 지지력에 맞춰 조정

lb = fz_min * ones(4,1);
ub = fz_max * ones(4,1);

%% QP initial guess
% 계산 시작점일 뿐, 목적함수의 참조값이 아님
x0 = total_mass * gravity / 4 * ones(4,1);
x0 = min(max(x0, lb), ub);

%% Force weights
% 순서: FL, FR, RL, RR
% 각 가중치는 양수로 설정
W = diag([1; 1; 1; 1]);

%% Solver 설정
options = optimoptions('quadprog', ...
    'Algorithm', 'active-set', ...
    'MaxIterations', 200);

%% 1단계
% minimize w'*w
%
% subject to
%   A*X - w = b
%   lb <= X <= ub
%
% 최적화 변수:
% z = [X_FL; X_FR; X_RL; X_RR; w_Fz; w_roll; w_pitch]

H1 = zeros(7,7);
H1(5:7,5:7) = 2 * eye(3);

f1 = zeros(7,1);

% A*X - w = b
Aeq1 = [A, -eye(3)];
beq1 = b;

% X에는 힘 제한, w에는 제한 없음
lb1 = [lb; -inf(3,1)];
ub1 = [ub;  inf(3,1)];

% 시작점도 등식을 만족하도록 설정
z0 = [x0; A*x0 - b];

[z_first, ~, flag1] = quadprog( ...
    H1, f1, ...
    [], [], ...
    Aeq1, beq1, ...
    lb1, ub1, z0, options);

if flag1 <= 0
    disp('QP stage 1 exitflag:');
    disp(flag1);
end

assert(flag1 > 0, 'Force QP stage 1 failed.');
assert(all(isfinite(z_first)), 'QP stage 1 is not finite.');

%% 1단계에서 달성한 결과
X_first = z_first(1:4);

% 실제 X_first가 만드는 wrench로 계산
b_achieved = A * X_first;
w_star = b_achieved - b;

%% 2단계
% minimize X'*X
%
% subject to
%   A*X = b_achieved
%   lb <= X <= ub
%
% 즉, 1단계의 최적 오차 w_star를 유지하면서
% 바퀴 힘의 제곱합만 최소화

H2 = 2 * eye(4);
f2 = zeros(4,1);

[X_final, ~, flag2] = quadprog( ...
    H2, f2, ...
    [], [], ...
    A, b_achieved, ...
    lb, ub, X_first, options);

if flag2 <= 0
    disp('QP stage 2 exitflag:');
    disp(flag2);
end

assert(flag2 > 0, 'Force QP stage 2 failed.');
assert(all(isfinite(X_final)), 'QP stage 2 is not finite.');

%% 출력: FL, FR, RL, RR의 Fz [N]
y = X_final;
end

== matlab function Katex_FullCar_R2017b_V03/DGIST/Attitude&Force distribution opt/GRF to Joint Torque/MATLAB Function ==
  data: u input; y output; sus_ang_fl input; sus_ang_fr input; sus_ang_rl input; sus_ang_rr input
function y = fcn(u, ...
    sus_ang_fl, sus_ang_fr, sus_ang_rl, sus_ang_rr)
% 입력
% u = [Fz_FL; Fz_FR; Fz_RL; Fz_RR] [N]
% sus_ang_* : XML 조인트 각도 [deg]
%
% 출력
% y = [tau_FL; tau_FR; tau_RL; tau_RR] [Nm]
% 각 서스펜션 motor에 전달할 토크

%% Input Setting
Fz = [u(1); u(2); u(3); u(4)];

theta = deg2rad([sus_ang_fl; sus_ang_fr; ...
                sus_ang_rl; sus_ang_rr]);

%% Robot
sus_link = 0.16;    % 서스펜션 링크 길이 [m]

sus_mass   = 2.5;  % 각 코너의 휠 제외 lumped mass [kg]
wheel_mass = 5.0;  % 각 휠 질량 [kg]

gravity = 1.67;    % XML 중력 크기 [m/s^2]

torque_limit = 100.0;  % gear=1인 현재 motor의 제한 [Nm]

%% Output Setting
y = zeros(4,1);

%% GRF to Joint Torque
for i = 1:4

    % 각도 변화에 따른 휠 중심의 z 위치 변화율 [m/rad]
    J_wheel = sus_link * cos(theta(i));

    % 각도 변화에 따른 서스펜션 COM의 z 위치 변화율
    J_sus = (sus_link/2) * cos(theta(i));

    % 서스펜션과 휠 무게에 대한 중력 보상 토크
    tau_gravity = ...
        J_sus   * sus_mass   * gravity ...
        + J_wheel * wheel_mass * gravity;

    % 목표 지면반력이 만드는 조인트 토크
    tau_contact = J_wheel * Fz(i);

    % MuJoCo motor에 필요한 토크
    tau_motor = tau_gravity - tau_contact;

    % 토크 제한
    y(i) = min(max(tau_motor, -torque_limit), torque_limit);

end

end

== matlab function Katex_FullCar_R2017b_V03/DGIST/_Reference_Generator/Slalom Profile/MATLAB Function ==
  data: t input; y output; f input; mag input; flag input
function y = fcn(t, f, mag, flag)

    % 상태 보존을 위한 persistent 변수 선언
    persistent current_f next_f current_mag next_mag t0 prev_phase

    if flag == 0
        % 초기화 상태: 출력 0과 함께 persistent 변수 초기화
        y = 0;
        current_f = f;    % 현재 사용 주파수를 입력 f로 설정
        next_f = f;       % 다음 주기 적용될 주파수도 우선 입력 f로 설정
        current_mag = mag;  % 현재 사용 진폭 설정
        next_mag = mag;     % 다음 주기 적용될 진폭도 우선 입력 mag로 설정
        t0 = t;            % 현재 시간을 주기의 시작 시간으로 저장
        prev_phase = 0;    % 이전 위상 값 초기화
    else  % flag == 1인 경우(정상 운용)
        % persistent 변수 초기화가 안된 경우 초기화 수행
        if isempty(current_f)
            current_f = f;
            next_f = f;
            current_mag = mag;
            next_mag = mag;
            t0 = t;
            prev_phase = 0;
        end

        % 주파수(f)와 진폭(mag)이 현재 주파수와 다르면 next_f와 next_mag에 저장
        if f ~= current_f
            next_f = f;
        end
        if mag ~= current_mag
            next_mag = mag;
        end

        % 현재 주기에서의 위상 계산: 현재 주파수(current_f)와 현재 진폭(current_mag)로 진행
        phase = 2 * pi * current_f * (t - t0);
        y = current_mag * sin(phase);  % 진폭을 고려하여 사인파 출력

        % 현재 위상의 modulo 계산 (0 ~ 2*pi 사이)
        current_mod = mod(phase, 2*pi);

        % 위상의 wrap-around 감지: 이전 위상(prev_phase)보다 작아진 경우 주기 종료
%         if current_mod < prev_phase
%             % 한 주기가 완료되었으므로, 다음 주기에는 next_f와 next_mag을 사용
%             current_f = next_f;
%             current_mag = next_mag;
%             t0 = t;  % 새로운 주기의 시작 시간 업데이트
%         end
        if current_mod < prev_phase
            % 현재 phase (랩 직전의 실제 위상)
            real_phase = 2*pi*current_f*(t - t0);
            % 새로운 주파수에 맞춰 phase continuity 보정
            t0 = t - real_phase/(2*pi*next_f);

            current_f   = next_f;
            current_mag = next_mag;
        end

        % 이전 위상 값 갱신
        prev_phase = current_mod;
    end
end

== matlab function Katex_FullCar_R2017b_V03/Scope/IMU/MATLAB Function ==
  data: q_in input; qout output
function qout = guardQuaternion(q_in)

persistent q_last

if isempty(q_last)
    q_last = [1.0;0.0;0.0;0.0];
end

q = reshape(q_in, 4, 1);
n2 = sum(q.*q);

if all(isfinite(q)) && isfinite(n2) && n2 > 1e-12
    q_last = q/ sqrt(n2);
end



qout = q_last;
end

== matlab function Katex_FullCar_R2017b_V03/DGIST/_High_Level_Ctrl/Chassis_FF_ctrl/Kinematic_Mapping_FF ==
  data: Vx_ref input; DriveVel_ref output; YawRate_ref input; L input; W input; WheelRadius input; SteerLimit input; SteerPos_ref output
function [DriveVel_ref, SteerPos_ref] = Kinematic_Mapping( ...
    Vx_ref, YawRate_ref, L, W, WheelRadius, SteerLimit)

%#codegen

% 출력 순서: FL, FR, RL, RR
DriveVel_ref = zeros(4,1);
SteerPos_ref = zeros(4,1);

% 안정성 판단 기준
Vx_stop_threshold = 0.01;       % [m/s]
YawRate_threshold = 1e-4;       % [rad/s]
Denominator_threshold = 1e-6;

% =========================================================
% Parameter 유효성 검사
% =========================================================
if L <= 0 || W < 0 || WheelRadius <= 0 || SteerLimit < 0
    return;
end

% =========================================================
% Safety 1: 정지 상태
% =========================================================
if abs(Vx_ref) < Vx_stop_threshold

    DriveVel_ref(:) = 0;
    SteerPos_ref(:) = 0;

    return;
end

% =========================================================
% Safety 2: 직진 상태
% =========================================================
if abs(YawRate_ref) < YawRate_threshold

    DriveVel_ref(:) = Vx_ref / WheelRadius;
    SteerPos_ref(:) = 0;

    return;
end

% =========================================================
% Chrono Kinematic Mapping
% =========================================================

% Rover 중심 ICR
rov_ICR = Vx_ref / YawRate_ref;

% 좌우 휠의 ICR 기준 거리
left_denominator  = rov_ICR - W/2;
right_denominator = rov_ICR + W/2;

% =========================================================
% Safety 3: 조향각 계산 분모 보호
% =========================================================
if abs(left_denominator) < Denominator_threshold

    if left_denominator < 0
        left_denominator = -Denominator_threshold;
    else
        left_denominator = Denominator_threshold;
    end
end

if abs(right_denominator) < Denominator_threshold

    if right_denominator < 0
        right_denominator = -Denominator_threshold;
    else
        right_denominator = Denominator_threshold;
    end
end

% =========================================================
% 각 Wheel ICR
% =========================================================
wheel_ICR = zeros(4,1);

wheel_ICR(1) = sqrt((L/2)^2 ...
                    + (rov_ICR-W/2)^2); % FL

wheel_ICR(2) = sqrt((L/2)^2 ...
                    + (rov_ICR+W/2)^2); % FR

wheel_ICR(3) = sqrt((L/2)^2 ...
                    + (rov_ICR-W/2)^2); % RL

wheel_ICR(4) = sqrt((L/2)^2 ...
                    + (rov_ICR+W/2)^2); % RR

% =========================================================
% Drive wheel angular velocity reference
% =========================================================
for i = 1:4

    DriveVel_ref(i) = ...
        (Vx_ref * abs(wheel_ICR(i)/abs(rov_ICR))) ...
        / WheelRadius;
end

% =========================================================
% Four-wheel steering position reference
% =========================================================
SteerPos_ref(1) = atan(( L/2)/left_denominator);  % FL
SteerPos_ref(2) = atan(( L/2)/right_denominator); % FR
SteerPos_ref(3) = atan((-L/2)/left_denominator);  % RL
SteerPos_ref(4) = atan((-L/2)/right_denominator); % RR

% =========================================================
% Steering angle saturation
% =========================================================
for i = 1:4

    if SteerPos_ref(i) > SteerLimit

        SteerPos_ref(i) = SteerLimit;

    elseif SteerPos_ref(i) < -SteerLimit

        SteerPos_ref(i) = -SteerLimit;
    end
end

end

== matlab function Katex_FullCar_R2017b_V03/DGIST/_Reference_Generator/Orientation Profile/MATLAB Function ==
  data: t input; y output; f input; mag input; flag input
function y = fcn(t, f, mag, flag)

    % 상태 보존을 위한 persistent 변수 선언
    persistent current_f next_f current_mag next_mag t0 prev_phase

    if flag == 0
        % 초기화 상태: 출력 0과 함께 persistent 변수 초기화
        y = 0;
        current_f = f;    % 현재 사용 주파수를 입력 f로 설정
        next_f = f;       % 다음 주기 적용될 주파수도 우선 입력 f로 설정
        current_mag = mag;  % 현재 사용 진폭 설정
        next_mag = mag;     % 다음 주기 적용될 진폭도 우선 입력 mag로 설정
        t0 = t;            % 현재 시간을 주기의 시작 시간으로 저장
        prev_phase = 0;    % 이전 위상 값 초기화
    else  % flag == 1인 경우(정상 운용)
        % persistent 변수 초기화가 안된 경우 초기화 수행
        if isempty(current_f)
            current_f = f;
            next_f = f;
            current_mag = mag;
            next_mag = mag;
            t0 = t;
            prev_phase = 0;
        end

        % 주파수(f)와 진폭(mag)이 현재 주파수와 다르면 next_f와 next_mag에 저장
        if f ~= current_f
            next_f = f;
        end
        if mag ~= current_mag
            next_mag = mag;
        end

        % 현재 주기에서의 위상 계산: 현재 주파수(current_f)와 현재 진폭(current_mag)로 진행
        phase = 2 * pi * current_f * (t - t0);
        y = current_mag * sin(phase);  % 진폭을 고려하여 사인파 출력

        % 현재 위상의 modulo 계산 (0 ~ 2*pi 사이)
        current_mod = mod(phase, 2*pi);

        % 위상의 wrap-around 감지: 이전 위상(prev_phase)보다 작아진 경우 주기 종료
%         if current_mod < prev_phase
%             % 한 주기가 완료되었으므로, 다음 주기에는 next_f와 next_mag을 사용
%             current_f = next_f;
%             current_mag = next_mag;
%             t0 = t;  % 새로운 주기의 시작 시간 업데이트
%         end
        if current_mod < prev_phase
            % 현재 phase (랩 직전의 실제 위상)
            real_phase = 2*pi*current_f*(t - t0);
            % 새로운 주파수에 맞춰 phase continuity 보정
            t0 = t - real_phase/(2*pi*next_f);

            current_f   = next_f;
            current_mag = next_mag;
        end

        % 이전 위상 값 갱신
        prev_phase = current_mod;
    end
end

== matlab function Katex_FullCar_R2017b_V03/DGIST/_Reference_Generator/Orientation Profile/MATLAB Function1 ==
  data: t input; y output; f input; mag input; flag input
function y = fcn(t, f, mag, flag)

    % 상태 보존을 위한 persistent 변수 선언
    persistent current_f next_f current_mag next_mag t0 prev_phase

    if flag == 0
        % 초기화 상태: 출력 0과 함께 persistent 변수 초기화
        y = 0;
        current_f = f;    % 현재 사용 주파수를 입력 f로 설정
        next_f = f;       % 다음 주기 적용될 주파수도 우선 입력 f로 설정
        current_mag = mag;  % 현재 사용 진폭 설정
        next_mag = mag;     % 다음 주기 적용될 진폭도 우선 입력 mag로 설정
        t0 = t;            % 현재 시간을 주기의 시작 시간으로 저장
        prev_phase = 0;    % 이전 위상 값 초기화
    else  % flag == 1인 경우(정상 운용)
        % persistent 변수 초기화가 안된 경우 초기화 수행
        if isempty(current_f)
            current_f = f;
            next_f = f;
            current_mag = mag;
            next_mag = mag;
            t0 = t;
            prev_phase = 0;
        end

        % 주파수(f)와 진폭(mag)이 현재 주파수와 다르면 next_f와 next_mag에 저장
        if f ~= current_f
            next_f = f;
        end
        if mag ~= current_mag
            next_mag = mag;
        end

        % 현재 주기에서의 위상 계산: 현재 주파수(current_f)와 현재 진폭(current_mag)로 진행
        phase = 2 * pi * current_f * (t - t0);
        y = current_mag * sin(phase);  % 진폭을 고려하여 사인파 출력

        % 현재 위상의 modulo 계산 (0 ~ 2*pi 사이)
        current_mod = mod(phase, 2*pi);

        % 위상의 wrap-around 감지: 이전 위상(prev_phase)보다 작아진 경우 주기 종료
%         if current_mod < prev_phase
%             % 한 주기가 완료되었으므로, 다음 주기에는 next_f와 next_mag을 사용
%             current_f = next_f;
%             current_mag = next_mag;
%             t0 = t;  % 새로운 주기의 시작 시간 업데이트
%         end
        if current_mod < prev_phase
            % 현재 phase (랩 직전의 실제 위상)
            real_phase = 2*pi*current_f*(t - t0);
            % 새로운 주파수에 맞춰 phase continuity 보정
            t0 = t - real_phase/(2*pi*next_f);

            current_f   = next_f;
            current_mag = next_mag;
        end

        % 이전 위상 값 갱신
        prev_phase = current_mod;
    end
end

== matlab function Katex_FullCar_R2017b_V03/DGIST/_High_Level_Ctrl/Chassis_FB_ctrl/Kinematic_Mapping_FB ==
  data: Vx_ref input; DriveVel_ref output; YawRate_ref input; L input; W input; WheelRadius input; SteerLimit input; SteerPos_ref output
function [DriveVel_ref, SteerPos_ref] = Kinematic_Mapping_FB( ...
    Vx_ref, YawRate_ref, L, W, WheelRadius, SteerLimit)

%#codegen

% 출력 순서: FL, FR, RL, RR
DriveVel_ref = zeros(4,1);
SteerPos_ref = zeros(4,1);

% 안정성 판단 기준
Vx_stop_threshold = 0.01;       % [m/s]
YawRate_threshold = 1e-4;       % [rad/s]
Denominator_threshold = 1e-6;

% =========================================================
% Parameter 유효성 검사
% =========================================================
if L <= 0 || W < 0 || WheelRadius <= 0 || SteerLimit < 0
    return;
end

% =========================================================
% Safety 1: 정지
% =========================================================
if abs(Vx_ref) < Vx_stop_threshold

    DriveVel_ref(:) = 0;
    SteerPos_ref(:) = 0;

    return;
end

% =========================================================
% Safety 2: 직진
% =========================================================
if abs(YawRate_ref) < YawRate_threshold

    % 전륜만 구동
    DriveVel_ref(1) = Vx_ref / WheelRadius; % FL
    DriveVel_ref(2) = Vx_ref / WheelRadius; % FR

    % 후륜은 passive wheel
    DriveVel_ref(3) = 0; % RL
    DriveVel_ref(4) = 0; % RR

    % 모든 조향각 0
    SteerPos_ref(:) = 0;

    return;
end

% =========================================================
% Front-wheel Kinematic Mapping
% =========================================================

% 후륜 차축 중심 기준 ICR
rov_ICR = Vx_ref / YawRate_ref;

left_denominator  = rov_ICR - W/2;
right_denominator = rov_ICR + W/2;

% =========================================================
% Safety 3: 조향각 분모 보호
% =========================================================
if abs(left_denominator) < Denominator_threshold

    if left_denominator < 0
        left_denominator = -Denominator_threshold;
    else
        left_denominator = Denominator_threshold;
    end
end

if abs(right_denominator) < Denominator_threshold

    if right_denominator < 0
        right_denominator = -Denominator_threshold;
    else
        right_denominator = Denominator_threshold;
    end
end

% =========================================================
% 전륜 Wheel ICR
% 기존 4WS: L/2
% 전륜 조향: L
% =========================================================
wheel_ICR_FL = sqrt(L^2 + (rov_ICR-W/2)^2);
wheel_ICR_FR = sqrt(L^2 + (rov_ICR+W/2)^2);

% =========================================================
% 전륜 Drive angular velocity reference
% =========================================================
DriveVel_ref(1) = ...
    (Vx_ref * abs(wheel_ICR_FL/abs(rov_ICR))) ...
    / WheelRadius; % FL

DriveVel_ref(2) = ...
    (Vx_ref * abs(wheel_ICR_FR/abs(rov_ICR))) ...
    / WheelRadius; % FR

% 후륜은 명령을 사용하지 않음
DriveVel_ref(3) = 0; % RL
DriveVel_ref(4) = 0; % RR

% =========================================================
% 전륜 Ackermann steering
% =========================================================
SteerPos_ref(1) = atan(L/left_denominator);  % FL
SteerPos_ref(2) = atan(L/right_denominator); % FR

% 후륜 조향각 0
SteerPos_ref(3) = 0; % RL
SteerPos_ref(4) = 0; % RR

% =========================================================
% 전륜 Steering saturation
% =========================================================
for i = 1:2

    if SteerPos_ref(i) > SteerLimit

        SteerPos_ref(i) = SteerLimit;

    elseif SteerPos_ref(i) < -SteerLimit

        SteerPos_ref(i) = -SteerLimit;
    end
end

end
